simulink model "sample"  (Simulink 10.3)
settings: Solver=VariableStepAuto  StartTime=0.0  StopTime=10.0  RelTol=1e-3
settings Model: Creator=VPQCONT  LastModifiedBy=VPQCONT  MultithreadedSim=on
settings DataIOCC: LimitDataPoints=on  SaveFormat=Dataset  SignalLoggingSaveFormat=Dataset  SaveOutput=off  SaveTime=off  ReturnWorkspaceOutputs=on
settings OptimizationCC: BlockReduction=off  BooleanDataType=off  ExpressionDepthLimit=128
settings DebuggingCC: SaveWithParameterizedLinksMsg=none  SignalResolutionControl=TryResolveAllWithWarning  FcnCallInpInsideContextMsg=error  AllowSymbolicDim=off  StateNameClashWarn=none
settings HardwareCC: ProdBitPerPointer=64  ProdBitPerSizeT=64  ProdBitPerPtrDiffT=64  ProdLargestAtomicFloat=Float  ProdIntDivRoundTo=Zero  ProdEndianess=LittleEndian  ProdWordSize=64  ProdHWDeviceType=Intel->x86-64 (Windows64)  TargetUnknown=on
settings ModelReferenceCC: PropagateSignalLabelsOutOfModel=on
settings GRTTargetCC: CombineOutputUpdateFcns=on  GRTInterface=off
settings ConfigComp: CovMetricSettings=dwe  CovSaveCumulativeToWorkspaceVar=off  CovSaveSingleToWorkspaceVar=off  CovExternalEMLEnable=on

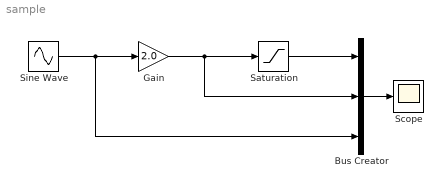
== system sample ==
  Bus Creator : BusCreator  Inputs=3
  Gain : Gain  Gain=2.0
  Saturation : Saturate
  Scope : Scope
  Sine Wave : Sin  SampleTime=0
  wires:
  Gain/1 -> Bus Creator/2, Saturation/1
  Sine Wave/1 -> Bus Creator/3, Gain/1
  Bus Creator/1 -> Scope/1
  Saturation/1 -> Bus Creator/1
